simulink model "closed_loop_model"  (R2019b)
settings: Solver=VariableStepAuto  StartTime=0.0  StopTime=400  RelTol=1e-3
libraries: simulink x2
settings Model: Creator=srikesh  LastModifiedBy=srikesh

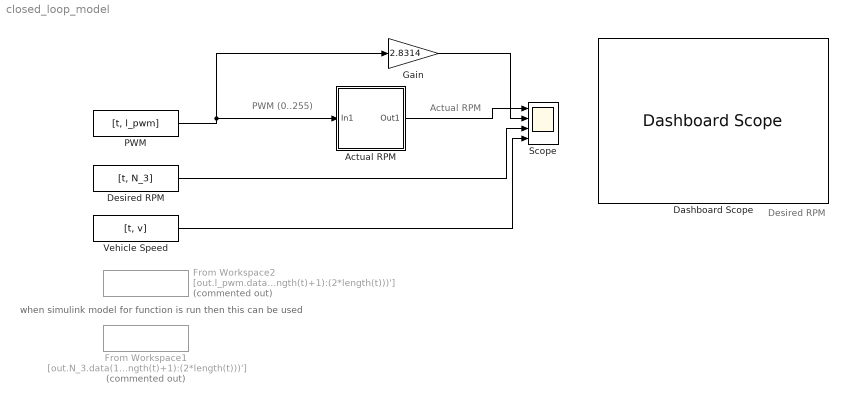
== system closed_loop_model ==
  note: Desired RPM
  note: PWM (0..255)
  note: when simulink model for function is run then this can be used
  note: Actual RPM
  Actual RPM : Subsystem
  Dashboard Scope : DashboardScope
  Desired RPM : FromWorkspace  VariableName=[t, N_3]  SampleTime=0
  From Workspace1 : FromWorkspace  Commented=on  VariableName=[out.N_3.data(1:length(t))', out.N_3.data((length(t)+1):(2*length(t)))']  SampleTime=0
  From Workspace2 : FromWorkspace  Commented=on  VariableName=[out.l_pwm.data(1:length(t))', out.l_pwm.data((length(t)+1):(2*length(t)))']  SampleTime=0
  Gain : Gain  Gain=2.8314
  PWM : FromWorkspace  VariableName=[t, l_pwm]  SampleTime=0
  Scope : Scope  NumInputPorts=4
  "Vehicle Speed " : FromWorkspace  VariableName=[t, v]  SampleTime=0
  wires:
  Desired RPM/1 -> Scope/3
  "Vehicle Speed "/1 -> Scope/4
  Actual RPM/1(Out1) -> Scope/1
  PWM/1 -> Gain/1, Actual RPM/1(In1)
  Gain/1 -> Scope/2

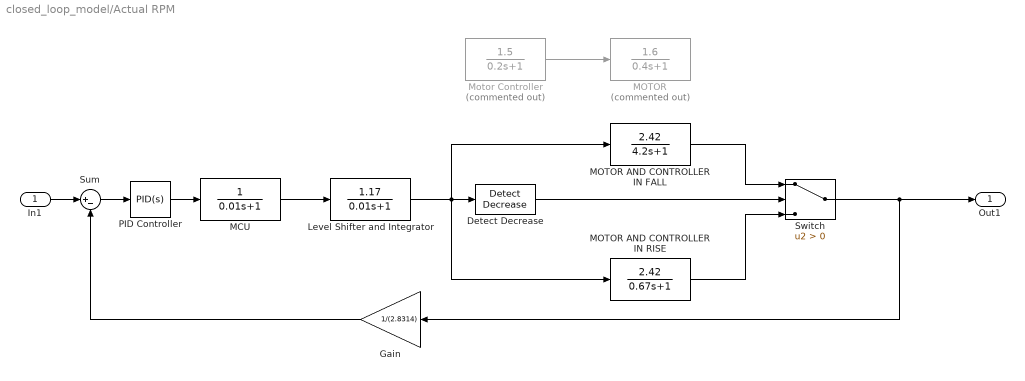
== system closed_loop_model/Actual RPM ==
  In1 : Inport
  Detect Decrease : simulink/Logic and Bit Operations/Detect Decrease  vinit=0.0  OutDataTypeStr=boolean
  Gain : Gain  Gain=1/(2.8314)
  Level Shifter and Integrator : TransferFcn  Numerator=[1.17]  Denominator=[0.01 1]
  MCU : TransferFcn  Denominator=[0.01 1]
  MOTOR : TransferFcn  Commented=on  Numerator=[1.6]  Denominator=[0.4 1]
  MOTOR AND CONTROLLER IN FALL : TransferFcn  Numerator=[2.42]  Denominator=[4.2 1]
  MOTOR AND CONTROLLER IN RISE : TransferFcn  Numerator=[2.42]  Denominator=[0.67 1]
  Motor Controller : TransferFcn  Commented=on  Numerator=[1.5]  Denominator=[0.2 1]
  PID Controller : simulink/Continuous/PID Controller  Controller=PID  Form=Parallel  TimeDomain=Continuous-time  SampleTime=-1  IntegratorMethod=Forward Euler  FilterMethod=Forward Euler  ControllerParametersSource=internal  P=15  I=0  D=0  UseFilter=on  N=100  TunerSelectOption=Transfer Function Based (PID Tuner App)  InitialConditionSource=internal  InitialConditionForIntegrator=0  InitialConditionForFilter=0  DifferentiatorICPrevScaledInput=0  ExternalReset=none  TrackingMode=off  Kt=1  LimitOutput=off  UpperSaturationLimit=inf  LowerSaturationLimit=-inf  LinearizeAsGain=on  AntiWindupMode=none  Kb=1  POutMin=[]  POutMax=[]  IOutMin=[]  IOutMax=[]  DOutMin=[]  DOutMax=[]  NOutMin=[]  NOutMax=[]  SumOutMin=[]  SumOutMax=[]  SaturationOutMin=[]  SaturationOutMax=[]  PParamMin=[]  PParamMax=[]  IParamMin=[]  IParamMax=[]  DParamMin=[]  DParamMax=[]  NParamMin=[]  NParamMax=[]  KbParamMin=[]  KbParamMax=[]  KtParamMin=[]  KtParamMax=[]  KbOutMin=[]  KbOutMax=[]  KtOutMin=[]  KtOutMax=[]  IntegratorOutMin=[]  IntegratorOutMax=[]  FilterOutMin=[]  FilterOutMax=[]  SumI1OutMin=[]  SumI1OutMax=[]  SumI2OutMin=[]  SumI2OutMax=[]  SumI3OutMin=[]  SumI3OutMax=[]  SumI4OutMin=[]  SumI4OutMax=[]  SumDOutMin=[]  SumDOutMax=[]  DifferentiatorOutMin=[]  DifferentiatorOutMax=[]  FilterDiffOutCoefMin=[]  FilterDiffOutCoefMax=[]  ReciprocalOutMin=[]  ReciprocalOutMax=[]  SumDenOutMin=[]  SumDenOutMax=[]  SumNumOutMin=[]  SumNumOutMax=[]  DivideOutMin=[]  DivideOutMax=[]  IntegratorContinuousStateAttributes=''  IntegratorStateMustResolveToSignalObject=off  IntegratorRTWStateStorageClass=Auto  FilterContinuousStateAttributes=''  FilterStateMustResolveToSignalObject=off  FilterRTWStateStorageClass=Auto  ParallelPVariant=InternalParameters  IdealPVariant=Disabled  IVariant=InternalParameters  DVariant=InternalParameters  IntegratorVariant=Continuous  SatVariant=Disabled  AWVariant=Passthrough  PCopyVariant=Disabled  TRVariant=Disabled  FdbkBlocksVariant=Forward  IdealPFdbkVariant=Disabled  SatFdbkVariant=Disabled  DerivativeFilterVariant=ContFilter  NVariant=InternalParameters  NCopyVariant=Disabled  FilterICVariant=InternalICsFilter  IntegratorICVariant=InternalICs  ExternalResetVariant=Disabled  TRSumVariant=Passthrough  SumFdbkVariant=Disabled  SumVariant=Sum_PID
  Sum : Sum  Inputs=|+-
  Switch : Switch  Criteria=u2 > Threshold
  Out1 : Outport
  wires:
  Motor Controller/1 -> MOTOR/1
  MCU/1 -> Level Shifter and Integrator/1
  Level Shifter and Integrator/1 -> MOTOR AND CONTROLLER IN RISE/1, MOTOR AND CONTROLLER IN FALL/1, Detect Decrease/1
  Detect Decrease/1 -> Switch/2
  MOTOR AND CONTROLLER IN FALL/1 -> Switch/1
  MOTOR AND CONTROLLER IN RISE/1 -> Switch/3
  Switch/1 -> Gain/1, Out1/1
  In1/1 -> Sum/1
  Sum/1 -> PID Controller/1
  PID Controller/1 -> MCU/1
  Gain/1 -> Sum/2
